simulink model "Beamforming"  (R2024b)
settings: Solver=FixedStepDiscrete  StartTime=0.0  StopTime=10.0  RelTol=1e-3
undefined symbols (not defined in the file): sysParams
settings Model: DataTypeOverride=Off  Creator=aless  LastModifiedBy=aless
settings SolverCC: PositivePriorityOrder=on
settings OptimizationCC: BlockReduction=off  ConditionallyExecuteInputs=off  DefaultParameterBehavior=Inlined  InheritOutputTypeSmallerThanSingle=on  EnhancedBackFolding=on  PassReuseOutputArgsAs=Individual arguments  ZeroExternalMemoryAtStartup=off  ZeroInternalMemoryAtStartup=off  MaxStackSize=64  OptimizeBlockOrder=speed  DifferentSizesBufferReuse=on  OptimizationCustomize=off  EfficientTunableParamExpr=on
settings DebuggingCC: AlgebraicLoopMsg=error  SingleTaskRateTransMsg=error  ParameterTunabilityLossMsg=error  UnconnectedInputMsg=warning  UnconnectedOutputMsg=warning  UnconnectedLineMsg=warning
settings HardwareCC: ProdBitPerPointer=32  ProdBitPerSizeT=32  ProdBitPerPtrDiffT=32  ProdLargestAtomicFloat=None  ProdIntDivRoundTo=Undefined  ProdEndianess=Unspecified  ProdWordSize=32  ProdHWDeviceType=ASIC/FPGA->ASIC/FPGA  TargetBitPerPointer=64  TargetBitPerSizeT=64  TargetBitPerPtrDiffT=64  TargetLongLongMode=on  TargetIntDivRoundTo=Zero  TargetEndianess=LittleEndian  TargetWordSize=64  TargetHWDeviceType=Custom Processor->MATLAB Host Computer  ProdEqTarget=off  HardwareBoardFeatureSet=SoCBlockset
settings ModelReferenceCC: ModelReferenceNumInstancesAllowed=Single
settings RTWCC: Description=Embedded Coder  SystemTargetFile=ert.tlc  HardwareBoard=Xilinx Zynq UltraScale+ RFSoC ZCU208 Evaluation Kit  TLCOptions="-aInlineSetEventsForThisBaseRateFcn=TLC_FALSE -aSuppressMultiTaskScheduler=TLC_FALSE  -aRateBasedStepFcn=0"  TemplateMakefile=ert_default_tmf  Toolchain=Linaro AArch64 Linux v6.3.1
settings CodeAppCC: ForceParamTrailComments=on  IgnoreCustomStorageClasses=off  OperatorAnnotations=on  SimulinkDataObjDesc=on  SFDataObjDesc=on  InsertBlockDesc=on

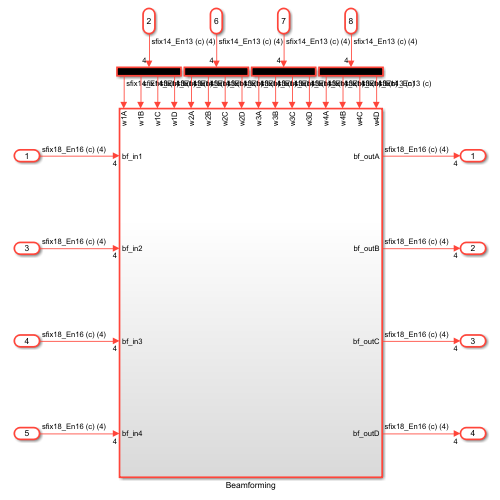
[thumbnail: Simulink's stored preview of the top-level diagram]
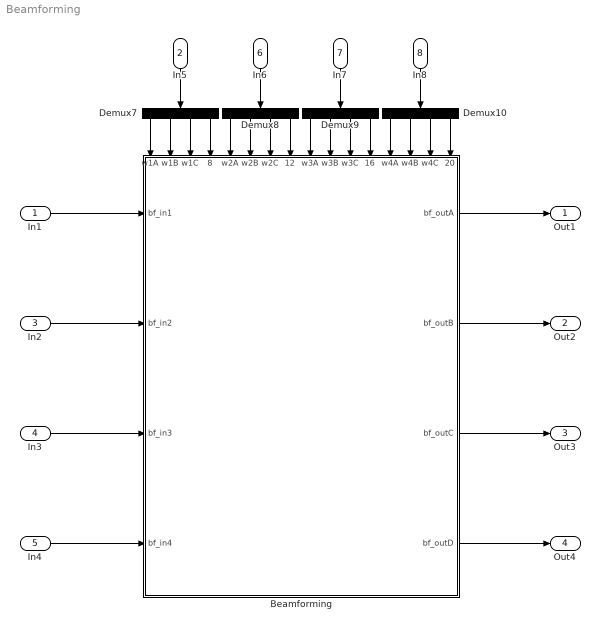
== system Beamforming ==
  In1 : Inport  PortDimensions=4  SampleTime=sysParams.FPGAClkPeriod
      settings: SignalType=complex
  In5 : Inport  Port=2  OutDataTypeStr=fixdt(1,14,13)  SampleTime=sysParams.FPGAClkPeriod
      settings: SignalType=complex
  In2 : Inport  Port=3  PortDimensions=4  SampleTime=sysParams.FPGAClkPeriod
      settings: SignalType=complex
  In3 : Inport  Port=4  PortDimensions=4  SampleTime=sysParams.FPGAClkPeriod
      settings: SignalType=complex
  In4 : Inport  Port=5  PortDimensions=4  SampleTime=sysParams.FPGAClkPeriod
      settings: SignalType=complex
  In6 : Inport  Port=6  OutDataTypeStr=fixdt(1,14,13)  SampleTime=sysParams.FPGAClkPeriod
      settings: SignalType=complex
  In7 : Inport  Port=7  OutDataTypeStr=fixdt(1,14,13)  SampleTime=sysParams.FPGAClkPeriod
      settings: SignalType=complex
  In8 : Inport  Port=8  OutDataTypeStr=fixdt(1,14,13)  SampleTime=sysParams.FPGAClkPeriod
      settings: SignalType=complex
  Beamforming : Subsystem
      settings: PortSchema="{\"entries\":[{\"content\":{\"sides\":[{\"content\":{\"connectorIds\":[\"In1\",\"In2\",\"In3\",\"In4\"]},\"type\":\"ConnectorPlacement.EquallySpacedRectSide\",\"uuid\":\"7b2ca850-5a44-4fe3-a571-bc89de8a8d8a\"},{\"content\":{\"connectorIds\":[\"Out1\",\"Out2\",\"Out3\",\"Out4\"],\"side\":\"RIGHT\"},\"type\":\"ConnectorPlacement.EquallySpacedRectSide\",\"uuid\":\"6a3de6dc-f4ee-4138-b8b6-8ad549f5ffcd\"},{\"content\":{\"connectorIds\":[\"In5\",\"In6\",\"In7\",\"In8\",\"In9\",\"In10\",\"In11\",\"In12\",\"In13\",\"In14\",\"In15\",\"In16\",\"In17\",\"In18\",\"In19\",\"In20\"],\"side\":\"TOP\"},\"type\":\"ConnectorPlacement.EquallySpacedRectSide\",\"uuid\":\"7b227388-a06d-4fee-a646-8c31054e6e12\"}]},\"type\":\"ConnectorPlacement.EquallySpacedConnector\",\"uuid\":\"7849fa84-ba55-4fcd-9e9c-b96e73e847f7\"}],\"packageUris\":[\"http://schema.mathworks.com/mf0/Connector/R2020b\"],\"version\":\"1.0\"}"
  Demux{7..10} (4 alike) : Demux
  Out1 : Outport
  Out2 : Outport  Port=2
  Out3 : Outport  Port=3
  Out4 : Outport  Port=4
  wires:
  Demux10/4 -> Beamforming/20(w4D)
  In2/1 -> Beamforming/2(bf_in2)
  Demux8/3 -> Beamforming/11(w2C)
  Demux7/1 -> Beamforming/5(w1A)
  Demux8/4 -> Beamforming/12(w2D)
  Demux10/2 -> Beamforming/18(w4B)
  Beamforming/1(bf_outA) -> Out1/1
  Beamforming/2(bf_outB) -> Out2/1
  In7/1 -> Demux9/1
  In8/1 -> Demux10/1
  Demux8/2 -> Beamforming/10(w2B)
  Demux9/4 -> Beamforming/16(w3D)
  Demux7/2 -> Beamforming/6(w1B)
  In1/1 -> Beamforming/1(bf_in1)
  In3/1 -> Beamforming/3(bf_in3)
  Beamforming/4(bf_outD) -> Out4/1
  Demux9/2 -> Beamforming/14(w3B)
  Demux7/4 -> Beamforming/8(w1D)
  Demux7/3 -> Beamforming/7(w1C)
  In4/1 -> Beamforming/4(bf_in4)
  Demux9/1 -> Beamforming/13(w3A)
  Beamforming/3(bf_outC) -> Out3/1
  In5/1 -> Demux7/1
  Demux8/1 -> Beamforming/9(w2A)
  Demux10/1 -> Beamforming/17(w4A)
  In6/1 -> Demux8/1
  Demux9/3 -> Beamforming/15(w3C)
  Demux10/3 -> Beamforming/19(w4C)

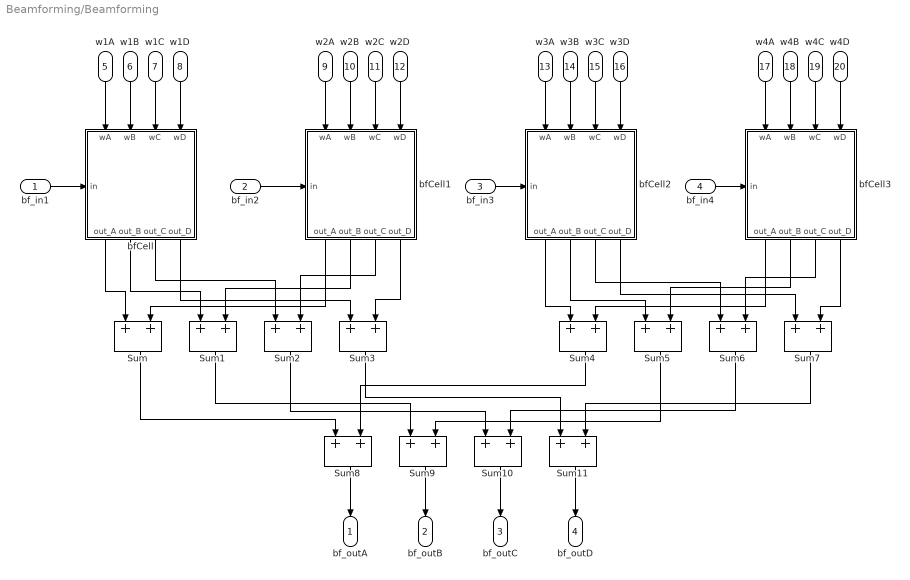
== system Beamforming/Beamforming ==
  bf_in1 : Inport
  bf_in2 : Inport  Port=2
  bf_in3 : Inport  Port=3
  bf_in4 : Inport  Port=4
  w1A : Inport  Port=5
  w1B : Inport  Port=6
  w1C : Inport  Port=7
  w1D : Inport  Port=8
  w2A : Inport  Port=9
  w2B : Inport  Port=10
  w2C : Inport  Port=11
  w2D : Inport  Port=12
  w3A : Inport  Port=13
  w3B : Inport  Port=14
  w3C : Inport  Port=15
  w3D : Inport  Port=16
  w4A : Inport  Port=17
  w4B : Inport  Port=18
  w4C : Inport  Port=19
  w4D : Inport  Port=20
  Sum{,1..11} (12 alike) : Sum  OutDataTypeStr=Inherit: Same as first input
  bfCell : Subsystem
      settings: PortSchema="{\"entries\":[{\"content\":{\"sides\":[{\"content\":{\"connectorIds\":[\"In1\",\"In2\",\"In3\",\"In4\"]},\"type\":\"ConnectorPlacement.EquallySpacedRectSide\",\"uuid\":\"0c826d6a-73c9-4dba-b1c5-31cfcef02303\"},{\"content\":{\"connectorIds\":[\"Out1\",\"Out2\",\"Out3\",\"Out4\"],\"side\":\"RIGHT\"},\"type\":\"ConnectorPlacement.EquallySpacedRectSide\",\"uuid\":\"e2d5e3de-4ff0-416d-bc8f-a95d356a0a64\"},{\"content\":{\"connectorIds\":[\"In5\"],\"side\":\"TOP\"},\"type\":\"ConnectorPlacement.EquallySpacedRectSide\",\"uuid\":\"bc2266f3-9c70-485a-9b9f-6558f87275cb\"}]},\"type\":\"ConnectorPlacement.EquallySpacedConnector\",\"uuid\":\"4675a578-71f2-44f5-ac97-67035b521010\"}],\"packageUris\":[\"http://schema.mathworks.com/mf0/Connector/R2020b\"],\"version\":\"1.0\"}"
  bfCell1 : Subsystem
      settings: PortSchema="{\"entries\":[{\"content\":{\"sides\":[{\"content\":{\"connectorIds\":[\"In1\",\"In2\",\"In3\",\"In4\"]},\"type\":\"ConnectorPlacement.EquallySpacedRectSide\",\"uuid\":\"0c826d6a-73c9-4dba-b1c5-31cfcef02303\"},{\"content\":{\"connectorIds\":[\"Out1\",\"Out2\",\"Out3\",\"Out4\"],\"side\":\"RIGHT\"},\"type\":\"ConnectorPlacement.EquallySpacedRectSide\",\"uuid\":\"e2d5e3de-4ff0-416d-bc8f-a95d356a0a64\"},{\"content\":{\"connectorIds\":[\"In5\"],\"side\":\"TOP\"},\"type\":\"ConnectorPlacement.EquallySpacedRectSide\",\"uuid\":\"bc2266f3-9c70-485a-9b9f-6558f87275cb\"}]},\"type\":\"ConnectorPlacement.EquallySpacedConnector\",\"uuid\":\"4675a578-71f2-44f5-ac97-67035b521010\"}],\"packageUris\":[\"http://schema.mathworks.com/mf0/Connector/R2020b\"],\"version\":\"1.0\"}"
  bfCell2 : Subsystem
      settings: PortSchema="{\"entries\":[{\"content\":{\"sides\":[{\"content\":{\"connectorIds\":[\"In1\",\"In2\",\"In3\",\"In4\"]},\"type\":\"ConnectorPlacement.EquallySpacedRectSide\",\"uuid\":\"0c826d6a-73c9-4dba-b1c5-31cfcef02303\"},{\"content\":{\"connectorIds\":[\"Out1\",\"Out2\",\"Out3\",\"Out4\"],\"side\":\"RIGHT\"},\"type\":\"ConnectorPlacement.EquallySpacedRectSide\",\"uuid\":\"e2d5e3de-4ff0-416d-bc8f-a95d356a0a64\"},{\"content\":{\"connectorIds\":[\"In5\"],\"side\":\"TOP\"},\"type\":\"ConnectorPlacement.EquallySpacedRectSide\",\"uuid\":\"bc2266f3-9c70-485a-9b9f-6558f87275cb\"}]},\"type\":\"ConnectorPlacement.EquallySpacedConnector\",\"uuid\":\"4675a578-71f2-44f5-ac97-67035b521010\"}],\"packageUris\":[\"http://schema.mathworks.com/mf0/Connector/R2020b\"],\"version\":\"1.0\"}"
  bfCell3 : Subsystem
      settings: PortSchema="{\"entries\":[{\"content\":{\"sides\":[{\"content\":{\"connectorIds\":[\"In1\",\"In2\",\"In3\",\"In4\"]},\"type\":\"ConnectorPlacement.EquallySpacedRectSide\",\"uuid\":\"0c826d6a-73c9-4dba-b1c5-31cfcef02303\"},{\"content\":{\"connectorIds\":[\"Out1\",\"Out2\",\"Out3\",\"Out4\"],\"side\":\"RIGHT\"},\"type\":\"ConnectorPlacement.EquallySpacedRectSide\",\"uuid\":\"e2d5e3de-4ff0-416d-bc8f-a95d356a0a64\"},{\"content\":{\"connectorIds\":[\"In5\"],\"side\":\"TOP\"},\"type\":\"ConnectorPlacement.EquallySpacedRectSide\",\"uuid\":\"bc2266f3-9c70-485a-9b9f-6558f87275cb\"}]},\"type\":\"ConnectorPlacement.EquallySpacedConnector\",\"uuid\":\"4675a578-71f2-44f5-ac97-67035b521010\"}],\"packageUris\":[\"http://schema.mathworks.com/mf0/Connector/R2020b\"],\"version\":\"1.0\"}"
  bf_outA : Outport
  bf_outB : Outport  Port=2
  bf_outC : Outport  Port=3
  bf_outD : Outport  Port=4
  wires:
  Sum8/1 -> bf_outA/1
  Sum9/1 -> bf_outB/1
  Sum10/1 -> bf_outC/1
  Sum11/1 -> bf_outD/1
  w1B/1 -> bfCell/2(wB)
  w1D/1 -> bfCell/4(wD)
  w1A/1 -> bfCell/1(wA)
  w1C/1 -> bfCell/3(wC)
  w2A/1 -> bfCell1/1(wA)
  w2B/1 -> bfCell1/2(wB)
  w2C/1 -> bfCell1/3(wC)
  w2D/1 -> bfCell1/4(wD)
  w3A/1 -> bfCell2/1(wA)
  w3B/1 -> bfCell2/2(wB)
  w3C/1 -> bfCell2/3(wC)
  w3D/1 -> bfCell2/4(wD)
  w4A/1 -> bfCell3/1(wA)
  w4B/1 -> bfCell3/2(wB)
  w4C/1 -> bfCell3/3(wC)
  w4D/1 -> bfCell3/4(wD)
  bf_in1/1 -> bfCell/5(in)
  bf_in2/1 -> bfCell1/5(in)
  bf_in3/1 -> bfCell2/5(in)
  bf_in4/1 -> bfCell3/5(in)
  bfCell/1(out_A) -> Sum/1
  bfCell1/1(out_A) -> Sum/2
  bfCell/2(out_B) -> Sum1/1
  bfCell1/2(out_B) -> Sum1/2
  bfCell/3(out_C) -> Sum2/1
  bfCell1/3(out_C) -> Sum2/2
  bfCell/4(out_D) -> Sum3/1
  bfCell1/4(out_D) -> Sum3/2
  bfCell2/1(out_A) -> Sum4/1
  bfCell3/1(out_A) -> Sum4/2
  bfCell2/2(out_B) -> Sum5/1
  bfCell3/2(out_B) -> Sum5/2
  bfCell2/3(out_C) -> Sum6/1
  bfCell3/3(out_C) -> Sum6/2
  bfCell2/4(out_D) -> Sum7/1
  bfCell3/4(out_D) -> Sum7/2
  Sum/1 -> Sum8/1
  Sum4/1 -> Sum8/2
  Sum1/1 -> Sum9/1
  Sum2/1 -> Sum10/1
  Sum5/1 -> Sum9/2
  Sum6/1 -> Sum10/2
  Sum3/1 -> Sum11/1
  Sum7/1 -> Sum11/2

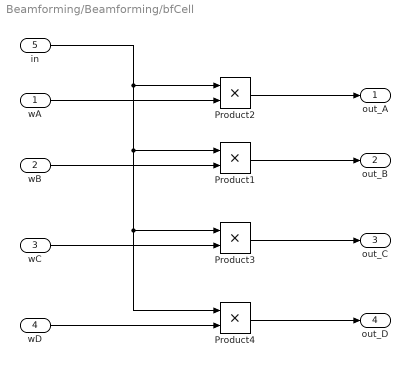
== system Beamforming/Beamforming/bfCell ==
  wA : Inport
  wB : Inport  Port=2
  wC : Inport  Port=3
  wD : Inport  Port=4
  in : Inport  Port=5
  Product{1..4} (4 alike) : Product  OutDataTypeStr=fixdt(1,FXP.sampWL,FXP.sampFL)
  out_A : Outport
  out_B : Outport  Port=2
  out_C : Outport  Port=3
  out_D : Outport  Port=4
  wires:
  wB/1 -> Product1/2
  in/1 -> Product2/1, Product1/1, Product4/1, Product3/1
  wC/1 -> Product3/2
  wD/1 -> Product4/2
  Product3/1 -> out_C/1
  Product1/1 -> out_B/1
  Product4/1 -> out_D/1
  Product2/1 -> out_A/1
  wA/1 -> Product2/2

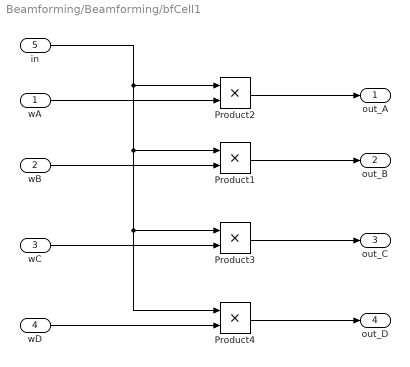
== system Beamforming/Beamforming/bfCell1 ==
  wA : Inport
  wB : Inport  Port=2
  wC : Inport  Port=3
  wD : Inport  Port=4
  in : Inport  Port=5
  Product{1..4} (4 alike) : Product  OutDataTypeStr=fixdt(1,FXP.sampWL,FXP.sampFL)
  out_A : Outport
  out_B : Outport  Port=2
  out_C : Outport  Port=3
  out_D : Outport  Port=4
  wires:
  wA/1 -> Product2/2
  Product2/1 -> out_A/1
  Product4/1 -> out_D/1
  Product1/1 -> out_B/1
  Product3/1 -> out_C/1
  wD/1 -> Product4/2
  wC/1 -> Product3/2
  in/1 -> Product3/1, Product4/1, Product1/1, Product2/1
  wB/1 -> Product1/2

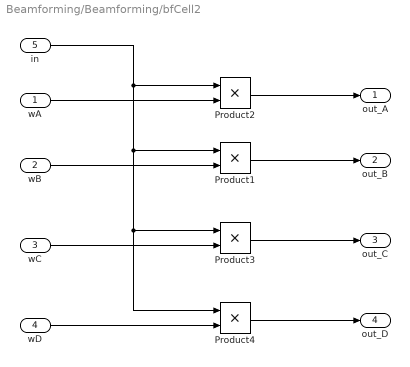
== system Beamforming/Beamforming/bfCell2 ==
  wA : Inport
  wB : Inport  Port=2
  wC : Inport  Port=3
  wD : Inport  Port=4
  in : Inport  Port=5
  Product{1..4} (4 alike) : Product  OutDataTypeStr=fixdt(1,FXP.sampWL,FXP.sampFL)
  out_A : Outport
  out_B : Outport  Port=2
  out_C : Outport  Port=3
  out_D : Outport  Port=4
  wires:
  wB/1 -> Product1/2
  in/1 -> Product2/1, Product1/1, Product4/1, Product3/1
  wC/1 -> Product3/2
  wD/1 -> Product4/2
  Product3/1 -> out_C/1
  Product1/1 -> out_B/1
  Product4/1 -> out_D/1
  Product2/1 -> out_A/1
  wA/1 -> Product2/2

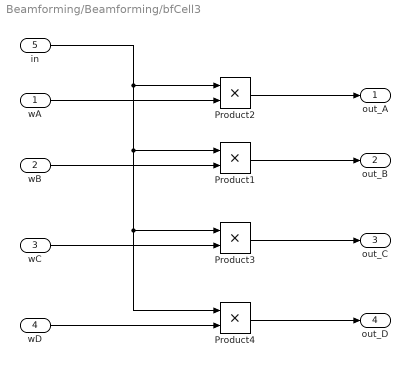
== system Beamforming/Beamforming/bfCell3 ==
  wA : Inport
  wB : Inport  Port=2
  wC : Inport  Port=3
  wD : Inport  Port=4
  in : Inport  Port=5
  Product{1..4} (4 alike) : Product  OutDataTypeStr=fixdt(1,FXP.sampWL,FXP.sampFL)
  out_A : Outport
  out_B : Outport  Port=2
  out_C : Outport  Port=3
  out_D : Outport  Port=4
  wires:
  wA/1 -> Product2/2
  Product2/1 -> out_A/1
  Product4/1 -> out_D/1
  Product1/1 -> out_B/1
  Product3/1 -> out_C/1
  wD/1 -> Product4/2
  wC/1 -> Product3/2
  in/1 -> Product3/1, Product4/1, Product1/1, Product2/1
  wB/1 -> Product1/2
